simulink model "HIL_comm"  (R2022a)
settings: Solver=FixedStepAuto  StartTime=0.0  StopTime=10.0  FixedStep=sim_TimeStep  RelTol=1e-3
undefined symbols (not defined in the file): param, param_vdc
libraries: instrumentseriallib x3, slrealtimeutilitieslib x2
settings Model: Creator=Usuario  LastModifiedBy=Usuario

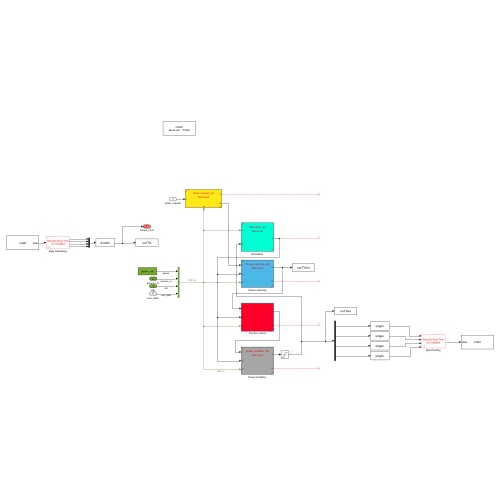
[thumbnail: Simulink's stored preview of the top-level diagram]
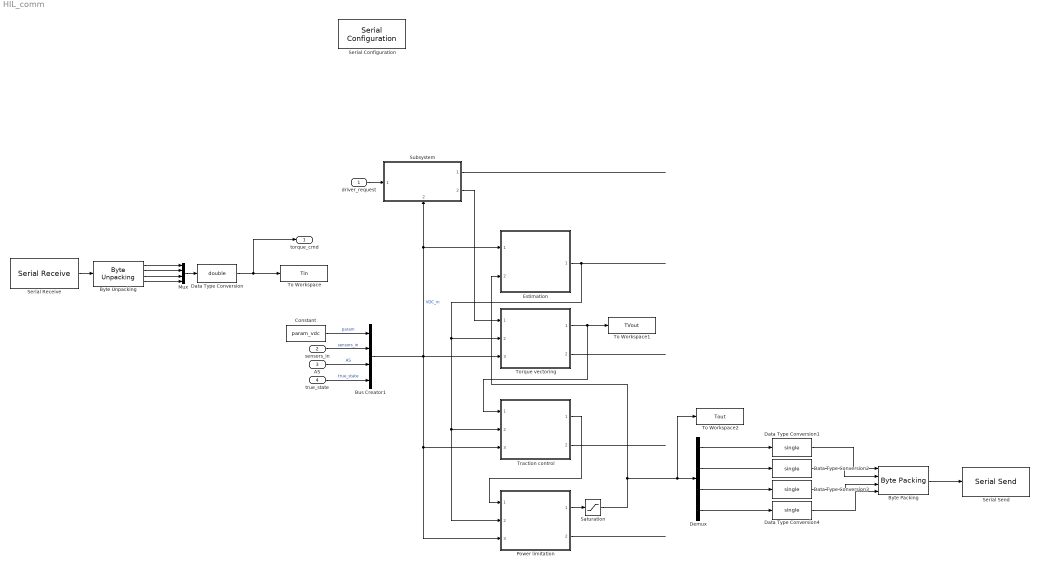
== system HIL_comm ==
  driver_request : Inport
  sensors_in : Inport  Port=2  OutDataTypeStr=Bus: sensorBus
  AS : Inport  Port=3
  true_state : Inport  Port=4  OutDataTypeStr=Bus: stateBus
  Bus Creator1 : BusCreator  Inputs=4
  Byte Packing : slrealtimeutilitieslib/Byte Packing  MaskPackedDataType=uint8  MaskUnpackedDataTypes={'single','single','single','single'}  MaskAlignment=1
  Byte Unpacking : slrealtimeutilitieslib/Byte Unpacking  MaskUnpackedDataTypes={'single','single','single','single'}  MaskUnpackedDataSizes={[1],[1],[1],[1]}  MaskAlignment=1
  Constant : Constant  Value=param_vdc  OutDataTypeStr=Bus: vdcBus
  Data Type Conversion : DataTypeConversion  OutDataTypeStr=double  SaturateOnIntegerOverflow=off  RndMeth=Floor
  Data Type Conversion{1..4} (4 alike) : DataTypeConversion  OutDataTypeStr=single  SaturateOnIntegerOverflow=off  RndMeth=Floor
  Demux : Demux
  Estimation : Subsystem  ReferencedSubsystem=Estimation_old
  Mux : Mux
  Power limitation : Subsystem  ReferencedSubsystem=Power_limitation_old
  Saturation : Saturate  UpperLimit=param.torque_limit_positive  LowerLimit=param.torque_limit_negative
  Serial Configuration : instrumentseriallib/Serial Configuration  Priority=-200000  PortSel=COM5  Port=COM5  ComPort=COM5  BaudRate=115200  DataBits=8  Parity=none  StopBits=1  ByteOrder=little-endian  FlowControl=none  Timeout=10  SimulateUsing=Interpreted execution  BlockInModel=on  aMode=1
  Serial Receive : instrumentseriallib/Serial Receive  Priority=1  PortSel=COM5  Port=COM5  ComPort=COM5  DataType=uint8  SaveDataType=uint8  ToggleHeader=on  Header=[171 205]  ToggleDataSize=on  DataSize=[16 1]  ToggleTerminator=off  Terminator=<none>  CustomTerminator=[]  InputFormat=Column major  EnableBlockingMode=on  ActionDataUnavailable=Output last received value  ActionWhenDataUnavailable=Output last received value  CustomValue=0  SampleTime=0.01  SimulateUsing=Interpreted execution  BlockInModel=on  aMode=1
  Serial Send : instrumentseriallib/Serial Send  Priority=1  PortSel=COM5  Port=COM5  ComPort=COM5  Header=[202 254]  Terminator=<none>  CustomTerminator=[]  EnableBlockingMode=off  SimulateUsing=Interpreted execution  BlockInModel=on  aMode=1
  Subsystem : Subsystem  ReferencedSubsystem=driver_request_old
      settings: PortSchema="{\"entries\":[{\"content\":{\"sides\":[{\"content\":{\"connectorIds\":[\"In1\"]},\"type\":\"ConnectorPlacement.EquallySpacedRectSide\",\"uuid\":\"6d0b78b3-ffc0-496d-8d3a-7ba3f556f803\"},{\"content\":{\"connectorIds\":[\"Out1\",\"Out2\"],\"side\":\"RIGHT\"},\"type\":\"ConnectorPlacement.EquallySpacedRectSide\",\"uuid\":\"be1dfba9-3592-437e-9363-a3609142bbc4\"},{\"content\":{\"connectorIds\":[],\"side\":\"TOP\"},\"type\":\"ConnectorPlacement.EquallySpacedRectSide\",\"uuid\":\"ddffd853-c46f-4213-b654-9451d95e6853\"},{\"content\":{\"connectorIds\":[\"In2\"],\"side\":\"BOTTOM\"},\"type\":\"ConnectorPlacement.EquallySpacedRectSide\",\"uuid\":\"b463dc20-ae30-4837-a1c3-1d0c4501f548\"}]},\"type\":\"ConnectorPlacement.EquallySpacedConnector\",\"uuid\":\"75a8dd9f-93ed-4a7a-b725-fd6938405663\"}],\"packageUris\":[\"http://schema.mathworks.com/mf0/Connector/R2020b\"],\"version\":\"1.0\"}"
  To Workspace : ToWorkspace  VariableName=Tin  SampleTime=-1
  To Workspace1 : ToWorkspace  VariableName=TVout  SaveFormat=Timeseries  SampleTime=-1
  To Workspace2 : ToWorkspace  VariableName=Tout  SampleTime=-1
  Torque vectoring : Subsystem  ReferencedSubsystem=Torque_vectoring_old
  Traction control : Subsystem  ReferencedSubsystem=Traction_control_old
  torque_cmd : Outport
  wires:
  Byte Packing/1 -> Serial Send/1
  Data Type Conversion/1 -> torque_cmd/1, To Workspace/1
  Data Type Conversion1/1 -> Byte Packing/1
  Byte Unpacking/4 -> Mux/4
  Mux/1 -> Data Type Conversion/1
  Byte Unpacking/3 -> Mux/3
  Byte Unpacking/2 -> Mux/2
  Byte Unpacking/1 -> Mux/1
  Serial Receive/1 -> Byte Unpacking/1
  Torque vectoring/2 -> ?
  Saturation/1 -> Estimation/2, To Workspace2/1, Demux/1
  Estimation/1 -> Torque vectoring/2, Traction control/2, Power limitation/2
  Subsystem/2 -> Torque vectoring/1
  true_state/1 -> Bus Creator1/4  "true_state"
  Traction control/1 -> Power limitation/1
  Power limitation/2 -> ?
  sensors_in/1 -> Bus Creator1/2  "sensors_in"
  AS/1 -> Bus Creator1/3  "AS"
  Subsystem/1 -> ?
  Torque vectoring/1 -> To Workspace1/1, Traction control/1
  Bus Creator1/1 -> Power limitation/3, Traction control/3, Subsystem/2, Estimation/1, Torque vectoring/3  "VDC_in"
  Power limitation/1 -> Saturation/1
  Constant/1 -> Bus Creator1/1  "param"
  Traction control/2 -> ?
  driver_request/1 -> Subsystem/1
  Demux/1 -> Data Type Conversion1/1
  Data Type Conversion2/1 -> Byte Packing/2
  Demux/2 -> Data Type Conversion2/1
  Data Type Conversion3/1 -> Byte Packing/3
  Demux/3 -> Data Type Conversion3/1
  Data Type Conversion4/1 -> Byte Packing/4
  Demux/4 -> Data Type Conversion4/1
